simulink model "sampleModel20"  (R2021a)
settings: Solver=VariableStepAuto  StartTime=0.0  StopTime=10.0  RelTol=1e-3
undefined symbols (not defined in the file): DiscIntNeverNeededParam, magnitude, Newton, Raphson
libraries: simulink x274, pid_lib x17
(part 7 of 16)

== system sampleModel20/cfblk93/cfblk6/cfblk8 ==
  cfblk1 : Inport
  cfblk5 : Inport  Port=2
  cfblk6 : Inport  Port=3
  cfblk7 : Inport  Port=4
  cfblk8 : Inport  Port=5
  cfblk9 : Inport  Port=6
  cfblk10 : Inport  Port=7
  cfblk3 : Math  Operator=hypot  SaturateOnIntegerOverflow=on
  cfblk4 : Sin  TimeSource=Use external signal  SampleTime=0
  cfblk2 : Outport
  wires:
  cfblk9/1 -> cfblk3/1
  cfblk1/1 -> cfblk3/2
  cfblk6/1 -> cfblk4/1
  cfblk10/1 -> cfblk2/1

== system sampleModel20/cfblk93/cfblk6/cfblk9 ==
  cfblk1 : Inport
  cfblk13 : Inport  Port=2
  cfblk14 : Inport  Port=3
  cfblk15 : Inport  Port=4
  cfblk16 : Inport  Port=5
  cfblk10 : Bias  Bias=[64527003.954944]
  cfblk11 : Subsystem
  cfblk12 : Subsystem
  cfblk17 : Delay  SampleTime=1
  cfblk18 : Delay  SampleTime=1
  cfblk3 : DiscreteIntegrator  ICPrevOutput=DiscIntNeverNeededParam  ICPrevScaledInput=DiscIntNeverNeededParam
  cfblk4 : Polyval  Coefs=[ +2.081618890e-019, -1.441693666e-014, +4.719686976e-010, -8.536869453e-006, +1.621573104e-001, -8.087801117e+001 ]
  cfblk5 : UnaryMinus
  cfblk6 : Polyval  Coefs=[ +2.081618890e-019, -1.441693666e-014, +4.719686976e-010, -8.536869453e-006, +1.621573104e-001, -8.087801117e+001 ]
  cfblk7 : Trigonometry
  cfblk8 : Math  Operator=mod  SaturateOnIntegerOverflow=on
  cfblk9 : MinMax  Function=max  Inputs=2
  cfblk2 : Outport
  wires:
  cfblk7/1 -> cfblk8/1
  cfblk10/1 -> cfblk7/1
  cfblk6/1 -> cfblk9/1
  cfblk8/1 -> cfblk3/1
  cfblk12/1(cfblk2) -> cfblk4/1
  cfblk13/1 -> cfblk5/1
  cfblk5/1 -> cfblk12/1(cfblk1)
  cfblk11/1(cfblk2) -> cfblk12/2(cfblk11)
  cfblk14/1 -> cfblk9/2, cfblk12/7(cfblk16)
  cfblk3/1 -> cfblk2/1, cfblk12/4(cfblk13)
  cfblk15/1 -> cfblk8/2, cfblk11/4(cfblk6)
  cfblk11/2(cfblk7) -> cfblk10/1, cfblk12/3(cfblk12)
  cfblk16/1 -> cfblk11/2(cfblk4), cfblk12/5(cfblk14), cfblk12/6(cfblk15)
  cfblk1/1 -> cfblk11/3(cfblk5)
  cfblk4/1 -> cfblk17/1
  cfblk17/1 -> cfblk11/1(cfblk1)
  cfblk9/1 -> cfblk18/1
  cfblk18/1 -> cfblk6/1

== system sampleModel20/cfblk93/cfblk7/cfblk10 ==
  cfblk1 : Inport
  cfblk6 : Inport  Port=2
  cfblk7 : Inport  Port=3
  cfblk3 : Sum
  cfblk4 : Subsystem
  cfblk5 : Subsystem
  cfblk8 : Delay  SampleTime=1
  cfblk9 : Delay  SampleTime=1
  cfblk2 : Outport
  wires:
  cfblk6/1 -> cfblk4/1(cfblk1), cfblk4/4(cfblk11), cfblk4/5(cfblk12), cfblk5/7(cfblk11)
  cfblk1/1 -> cfblk3/1, cfblk5/4(cfblk8), cfblk5/5(cfblk9)
  cfblk3/1 -> cfblk4/2(cfblk9), cfblk5/6(cfblk10), cfblk4/6(cfblk13)
  cfblk5/1(cfblk2) -> cfblk2/1, cfblk9/1
  cfblk7/1 -> cfblk5/1(cfblk1), cfblk4/7(cfblk14), cfblk4/8(cfblk15)
  cfblk4/2(cfblk16) -> cfblk5/2(cfblk6)
  cfblk4/3(cfblk17) -> cfblk5/3(cfblk7)
  cfblk4/1(cfblk2) -> cfblk8/1
  cfblk8/1 -> cfblk3/2
  cfblk9/1 -> cfblk4/3(cfblk10)

== system sampleModel20/cfblk94/cfblk10/cfblk6 ==
  cfblk1 : Inport
  cfblk6 : Inport  Port=2
  cfblk7 : Inport  Port=3
  cfblk8 : Inport  Port=4
  cfblk9 : Inport  Port=5
  cfblk10 : Inport  Port=6
  cfblk3 : simulink/Discrete/Tapped Delay  vinit=0.0  samptime=-1  NumDelays=1  DelayOrder=Oldest  includeCurrent=off
  cfblk4 : Sqrt  SaturateOnIntegerOverflow=on
  cfblk5 : Subsystem
  cfblk2 : Outport
  cfblk11 : Outport  Port=2
  cfblk12 : Outport  Port=3
  cfblk13 : Outport  Port=4
  wires:
  cfblk6/1 -> cfblk5/1(cfblk1)
  cfblk8/1 -> cfblk12/1
  cfblk3/1 -> cfblk5/2(cfblk5)
  cfblk10/1 -> cfblk13/1
  cfblk9/1 -> cfblk3/1, cfblk5/4(cfblk7)
  cfblk4/1 -> cfblk11/1
  cfblk5/1(cfblk2) -> cfblk2/1
  cfblk7/1 -> cfblk4/1
  cfblk1/1 -> cfblk5/3(cfblk6), cfblk5/5(cfblk8)

== system sampleModel20/cfblk94/cfblk10/cfblk7 ==
  cfblk1 : Inport
  cfblk10 : Inport  Port=2
  cfblk11 : Inport  Port=3
  cfblk12 : Inport  Port=4
  cfblk13 : Inport  Port=5
  cfblk{15..26} (12 alike) : Delay  SampleTime=1
  cfblk3 : ComplexToMagnitudeAngle
  cfblk4 : Subsystem
  cfblk5 : Subsystem
  cfblk6 : Subsystem
  cfblk7 : Subsystem
  cfblk8 : Subsystem
  cfblk9 : Subsystem
  cfblk2 : Outport
  cfblk14 : Outport  Port=2
  wires:
  cfblk1/1 -> cfblk8/1(cfblk1), cfblk4/5(cfblk10)
  cfblk8/1(cfblk2) -> cfblk5/1(cfblk1)
  cfblk6/1(cfblk2) -> cfblk2/1
  cfblk9/1(cfblk2) -> cfblk3/1
  cfblk12/1 -> cfblk9/2(cfblk10), cfblk7/6(cfblk14)
  cfblk13/1 -> cfblk5/2(cfblk11), cfblk6/4(cfblk12), cfblk8/7(cfblk9), cfblk7/8(cfblk16)
  cfblk3/2 -> cfblk4/8(cfblk13), cfblk16/1, cfblk17/1, cfblk18/1, cfblk19/1
  cfblk8/2(cfblk10) -> cfblk7/1(cfblk1)
  cfblk11/1 -> cfblk7/3(cfblk11), cfblk4/1(cfblk1), cfblk4/2(cfblk7), cfblk7/5(cfblk13), cfblk4/6(cfblk11)
  cfblk4/1(cfblk2) -> cfblk14/1
  cfblk9/3(cfblk17) -> cfblk21/1, cfblk22/1, cfblk23/1
  cfblk8/3(cfblk11) -> cfblk5/3(cfblk12)
  cfblk7/1(cfblk2) -> cfblk6/1(cfblk1)
  cfblk7/2(cfblk17) -> cfblk6/2(cfblk10), cfblk4/9(cfblk14), cfblk24/1, cfblk25/1
  cfblk10/1 -> cfblk5/4(cfblk13)
  cfblk6/2(cfblk14) -> cfblk9/4(cfblk12), cfblk4/3(cfblk8), cfblk9/7(cfblk15)
  cfblk5/1(cfblk2) -> cfblk7/4(cfblk12)
  cfblk5/2(cfblk16) -> cfblk6/3(cfblk11)
  cfblk5/3(cfblk17) -> cfblk9/5(cfblk13), cfblk4/4(cfblk9), cfblk9/6(cfblk14), cfblk4/7(cfblk12), cfblk26/1
  cfblk3/1 -> cfblk15/1
  cfblk15/1 -> cfblk9/1(cfblk1)
  cfblk16/1 -> cfblk9/3(cfblk11)
  cfblk17/1 -> cfblk5/6(cfblk15)
  cfblk18/1 -> cfblk6/5(cfblk13)
  cfblk19/1 -> cfblk7/7(cfblk15)
  cfblk9/2(cfblk16) -> cfblk20/1
  cfblk20/1 -> cfblk7/2(cfblk10)
  cfblk21/1 -> cfblk8/2(cfblk4)
  cfblk22/1 -> cfblk8/3(cfblk5)
  cfblk23/1 -> cfblk8/4(cfblk6)
  cfblk24/1 -> cfblk5/5(cfblk14)
  cfblk25/1 -> cfblk8/6(cfblk8)
  cfblk26/1 -> cfblk8/5(cfblk7)

== system sampleModel20/cfblk94/cfblk11/cfblk6 ==
  cfblk1 : Inport
  cfblk6 : Inport  Port=2
  cfblk7 : Inport  Port=3
  cfblk8 : Inport  Port=4
  cfblk9 : Inport  Port=5
  cfblk10 : Delay  SampleTime=1
  cfblk11 : Delay  SampleTime=1
  cfblk12 : Delay  SampleTime=1
  cfblk3 : Delay  DelayLengthSource=Input port  SampleTime=1
      settings: InputPortMap=u0,p1
  cfblk4 : Subsystem
  cfblk5 : Subsystem
  cfblk2 : Outport
  wires:
  cfblk3/1 -> cfblk5/1(cfblk1)
  cfblk8/1 -> cfblk4/1(cfblk1)
  cfblk6/1 -> cfblk2/1
  cfblk4/1(cfblk2) -> cfblk5/2(cfblk4)
  cfblk1/1 -> cfblk4/3(cfblk10)
  cfblk9/1 -> cfblk3/1, cfblk4/6(cfblk13)
  cfblk4/2(cfblk14) -> cfblk3/2
  cfblk7/1 -> cfblk5/3(cfblk5)
  cfblk4/3(cfblk15) -> cfblk5/4(cfblk6)
  cfblk5/1(cfblk2) -> cfblk10/1
  cfblk10/1 -> cfblk4/2(cfblk9)
  cfblk5/2(cfblk7) -> cfblk11/1
  cfblk11/1 -> cfblk4/4(cfblk11)
  cfblk5/3(cfblk8) -> cfblk12/1
  cfblk12/1 -> cfblk4/5(cfblk12)

== system sampleModel20/cfblk94/cfblk11/cfblk7 ==
  cfblk1 : Inport
  cfblk6 : Inport  Port=2
  cfblk3 : MinMax  Inputs=2
  cfblk4 : Subsystem
  cfblk5 : Subsystem
  cfblk8 : Delay  SampleTime=1
  cfblk9 : Delay  SampleTime=1
  cfblk2 : Outport
  cfblk7 : Outport  Port=2
  wires:
  cfblk3/1 -> cfblk7/1, cfblk5/1(cfblk1), cfblk5/3(cfblk10)
  cfblk6/1 -> cfblk4/1(cfblk1), cfblk5/2(cfblk9)
  cfblk5/1(cfblk2) -> cfblk4/2(cfblk8), cfblk4/4(cfblk10)
  cfblk4/1(cfblk2) -> cfblk8/1, cfblk9/1
  cfblk1/1 -> cfblk2/1, cfblk3/2, cfblk4/3(cfblk9)
  cfblk8/1 -> cfblk3/1
  cfblk9/1 -> cfblk5/4(cfblk11)

== system sampleModel20/cfblk94/cfblk6/cfblk7 ==
  cfblk1 : Inport
  cfblk9 : Inport  Port=2
  cfblk10 : Inport  Port=3
  cfblk11 : Inport  Port=4
  cfblk{12..18} (7 alike) : Delay  SampleTime=1
  cfblk3 : Sin  TimeSource=Use external signal  SampleTime=0
  cfblk4 : Product  Inputs=*
  cfblk5 : Subsystem
  cfblk6 : Subsystem
  cfblk7 : Subsystem
  cfblk8 : Subsystem
  cfblk2 : Outport
  wires:
  cfblk11/1 -> cfblk4/1, cfblk3/1, cfblk8/6(cfblk11), cfblk5/7(cfblk11)
  cfblk1/1 -> cfblk6/1(cfblk1)
  cfblk3/1 -> cfblk7/1(cfblk1), cfblk6/8(cfblk14), cfblk5/6(cfblk10)
  cfblk7/1(cfblk2) -> cfblk2/1
  cfblk9/1 -> cfblk6/2(cfblk8), cfblk5/2(cfblk6), cfblk7/4(cfblk12), cfblk7/6(cfblk14), cfblk7/8(cfblk16)
  cfblk7/2(cfblk17) -> cfblk15/1, cfblk16/1, cfblk17/1, cfblk18/1
  cfblk4/1 -> cfblk7/2(cfblk10), cfblk7/7(cfblk15)
  cfblk6/1(cfblk2) -> cfblk8/3(cfblk8)
  cfblk10/1 -> cfblk6/5(cfblk11), cfblk7/5(cfblk13), cfblk5/4(cfblk8)
  cfblk8/3(cfblk15) -> cfblk5/1(cfblk1), cfblk7/3(cfblk11)
  cfblk6/2(cfblk15) -> cfblk8/4(cfblk9), cfblk5/3(cfblk7), cfblk8/7(cfblk12), cfblk8/8(cfblk13), cfblk5/5(cfblk9)
  cfblk8/1(cfblk2) -> cfblk12/1
  cfblk12/1 -> cfblk6/3(cfblk9)
  cfblk8/2(cfblk14) -> cfblk13/1
  cfblk13/1 -> cfblk6/4(cfblk10)
  cfblk5/1(cfblk2) -> cfblk14/1
  cfblk14/1 -> cfblk8/1(cfblk1)
  cfblk15/1 -> cfblk8/2(cfblk7)
  cfblk16/1 -> cfblk6/6(cfblk12)
  cfblk17/1 -> cfblk8/5(cfblk10)
  cfblk18/1 -> cfblk6/7(cfblk13)

== system sampleModel20/cfblk94/cfblk6/cfblk8 ==
  cfblk1 : Inport
  cfblk9 : Inport  Port=2
  cfblk10 : Inport  Port=3
  cfblk11 : Inport  Port=4
  cfblk12 : Inport  Port=5
  cfblk13 : Inport  Port=6
  cfblk{14..23} (10 alike) : Delay  SampleTime=1
  cfblk3 : Assignment  DiagnosticForDimensions=Warning  IndexOptions=Index vector (dialog)  Indices=1  OutputSizes=1
  cfblk4 : Assignment  DiagnosticForDimensions=Warning  IndexOptions=Index vector (dialog)  Indices=1  OutputSizes=1
  cfblk5 : Subsystem
  cfblk6 : Subsystem
  cfblk7 : Subsystem
  cfblk8 : Subsystem
  cfblk2 : Outport
  wires:
  cfblk9/1 -> cfblk4/1
  cfblk3/1 -> cfblk2/1, cfblk15/1, cfblk16/1
  cfblk12/1 -> cfblk4/2, cfblk6/7(cfblk14), cfblk8/6(cfblk10)
  cfblk4/1 -> cfblk6/1(cfblk1)
  cfblk13/1 -> cfblk7/1(cfblk1), cfblk7/2(cfblk9)
  cfblk8/1(cfblk2) -> cfblk5/1(cfblk1)
  cfblk10/1 -> cfblk5/2(cfblk9)
  cfblk11/1 -> cfblk3/1, cfblk7/3(cfblk10), cfblk7/4(cfblk11)
  cfblk1/1 -> cfblk8/2(cfblk6), cfblk8/4(cfblk8), cfblk5/8(cfblk15), cfblk7/6(cfblk13)
  cfblk7/4(cfblk16) -> cfblk21/1, cfblk22/1
  cfblk6/1(cfblk2) -> cfblk3/2
  cfblk8/2(cfblk11) -> cfblk6/4(cfblk11)
  cfblk5/2(cfblk16) -> cfblk6/5(cfblk12), cfblk6/6(cfblk13), cfblk23/1
  cfblk6/2(cfblk15) -> cfblk7/5(cfblk12), cfblk17/1
  cfblk5/1(cfblk2) -> cfblk14/1
  cfblk14/1 -> cfblk8/3(cfblk7)
  cfblk15/1 -> cfblk5/5(cfblk12)
  cfblk16/1 -> cfblk5/7(cfblk14)
  cfblk17/1 -> cfblk5/4(cfblk11)
  cfblk7/1(cfblk2) -> cfblk18/1
  cfblk18/1 -> cfblk6/2(cfblk9)
  cfblk7/2(cfblk14) -> cfblk19/1
  cfblk19/1 -> cfblk6/3(cfblk10)
  cfblk7/3(cfblk15) -> cfblk20/1
  cfblk20/1 -> cfblk8/1(cfblk1)
  cfblk21/1 -> cfblk5/3(cfblk10)
  cfblk22/1 -> cfblk5/6(cfblk13)
  cfblk23/1 -> cfblk8/5(cfblk9)

== system sampleModel20/cfblk94/cfblk7/cfblk4 ==
  cfblk1 : Inport
  cfblk10 : Inport  Port=2
  cfblk11 : Inport  Port=3
  cfblk{13..18} (6 alike) : Delay  SampleTime=1
  cfblk3 : Product  Inputs=**
  cfblk4 : Polyval  Coefs=[ +2.081618890e-019, -1.441693666e-014, +4.719686976e-010, -8.536869453e-006, +1.621573104e-001, -8.087801117e+001 ]
  cfblk5 : Subsystem
  cfblk6 : Subsystem
  cfblk7 : Subsystem
  cfblk8 : Subsystem
  cfblk9 : Subsystem
  cfblk2 : Outport
  cfblk12 : Outport  Port=2
  wires:
  cfblk3/1 -> cfblk8/5(cfblk7), cfblk18/1
  cfblk9/1(cfblk2) -> cfblk4/1, cfblk8/2(cfblk4), cfblk8/3(cfblk5), cfblk2/1, cfblk7/2(cfblk7)
  cfblk10/1 -> cfblk3/1, cfblk8/8(cfblk10)
  cfblk1/1 -> cfblk6/3(cfblk12)
  cfblk7/1(cfblk2) -> cfblk5/1(cfblk1)
  cfblk6/1(cfblk2) -> cfblk9/1(cfblk1)
  cfblk8/2(cfblk11) -> cfblk7/1(cfblk1)
  cfblk6/2(cfblk17) -> cfblk3/2, cfblk7/3(cfblk8), cfblk7/4(cfblk9), cfblk8/4(cfblk6), cfblk8/6(cfblk8), cfblk8/7(cfblk9)
  cfblk11/1 -> cfblk9/3(cfblk9), cfblk6/7(cfblk16)
  cfblk5/2(cfblk8) -> cfblk12/1
  cfblk7/3(cfblk11) -> cfblk5/2(cfblk7), cfblk16/1
  cfblk4/1 -> cfblk8/1(cfblk1)
  cfblk8/1(cfblk2) -> cfblk13/1
  cfblk13/1 -> cfblk6/2(cfblk11)
  cfblk5/1(cfblk2) -> cfblk14/1
  cfblk14/1 -> cfblk6/4(cfblk13)
  cfblk7/2(cfblk10) -> cfblk15/1
  cfblk15/1 -> cfblk9/2(cfblk8)
  cfblk16/1 -> cfblk6/5(cfblk14)
  cfblk8/3(cfblk12) -> cfblk17/1
  cfblk17/1 -> cfblk6/6(cfblk15)
  cfblk18/1 -> cfblk6/1(cfblk1)

== system sampleModel20/cfblk94/cfblk8/cfblk8 ==
  cfblk1 : Inport
  cfblk8 : Inport  Port=2
  cfblk9 : Inport  Port=3
  cfblk11 : Delay  SampleTime=1
  cfblk3 : Sum  Inputs=+
  cfblk4 : Sum  Inputs=+
  cfblk5 : MinMax  Function=max
  cfblk6 : Subsystem
  cfblk7 : Subsystem
  cfblk2 : Outport
  cfblk10 : Outport  Port=2
  wires:
  cfblk6/1(cfblk2) -> cfblk5/1, cfblk7/4(cfblk9), cfblk7/7(cfblk12)
  cfblk5/1 -> cfblk7/1(cfblk1)
  cfblk9/1 -> cfblk3/1
  cfblk4/1 -> cfblk2/1, cfblk11/1
  cfblk3/1 -> cfblk7/2(cfblk7), cfblk6/3(cfblk12), cfblk7/5(cfblk10), cfblk10/1, cfblk7/6(cfblk11)
  cfblk1/1 -> cfblk6/2(cfblk11)
  cfblk8/1 -> cfblk7/3(cfblk8)
  cfblk7/1(cfblk2) -> cfblk4/1
  cfblk11/1 -> cfblk6/1(cfblk1)

== system sampleModel20/cfblk94/cfblk8/cfblk9 ==
  cfblk1 : Inport
  cfblk6 : Inport  Port=2
  cfblk7 : Inport  Port=3
  cfblk8 : Inport  Port=4
  cfblk3 : Squeeze
  cfblk4 : simulink/Math Operations/MinMax Running Resettable  Function=min  vinit=0.0
  cfblk5 : Subsystem
  cfblk2 : Outport
  cfblk9 : Outport  Port=2
  wires:
  cfblk1/1 -> cfblk5/1(cfblk1)
  cfblk3/1 -> cfblk5/2(cfblk6), cfblk5/5(cfblk9)
  cfblk6/1 -> cfblk4/1, cfblk5/3(cfblk7)
  cfblk8/1 -> cfblk4/2
  cfblk7/1 -> cfblk2/1
  cfblk5/1(cfblk2) -> cfblk9/1
  cfblk4/1 -> cfblk3/1, cfblk5/4(cfblk8), cfblk5/6(cfblk10)

== system sampleModel20/cfblk94/cfblk9/cfblk6 ==
  cfblk1 : Inport
  cfblk11 : Inport  Port=2
  cfblk12 : Inport  Port=3
  cfblk10 : Subsystem
  cfblk{15..21} (7 alike) : Delay  SampleTime=1
  cfblk3 : Gain  Gain=[597722013.813151]
  cfblk4 : Gain  Gain=[-468579084.699582]
  cfblk5 : simulink/Math Operations/Slider Gain  gain=1  low=0  high=2
  cfblk6 : ComplexToMagnitudeAngle
  cfblk7 : DotProduct  InputSameDT=on  OutDataTypeStr=Inherit: Inherit via internal rule
  cfblk8 : Subsystem
  cfblk9 : Subsystem
  cfblk2 : Outport
  cfblk13 : Outport  Port=2
  cfblk14 : Outport  Port=3
  wires:
  cfblk3/1 -> cfblk5/1, cfblk10/5(cfblk6), cfblk10/8(cfblk9)
  cfblk10/1(cfblk2) -> cfblk13/1
  cfblk11/1 -> cfblk6/1, cfblk10/2(cfblk3), cfblk10/4(cfblk5)
  cfblk5/1 -> cfblk2/1, cfblk10/3(cfblk4), cfblk15/1
  cfblk6/1 -> cfblk9/1(cfblk1)
  cfblk10/2(cfblk12) -> cfblk7/2
  cfblk8/1(cfblk2) -> cfblk3/1
  cfblk10/3(cfblk13) -> cfblk14/1
  cfblk12/1 -> cfblk8/2(cfblk9)
  cfblk6/2 -> cfblk9/2(cfblk7)
  cfblk7/1 -> cfblk9/3(cfblk8), cfblk20/1
  cfblk1/1 -> cfblk8/3(cfblk10), cfblk10/6(cfblk7), cfblk10/7(cfblk8)
  cfblk9/1(cfblk2) -> cfblk4/1
  cfblk8/2(cfblk13) -> cfblk9/4(cfblk9)
  cfblk9/3(cfblk11) -> cfblk18/1, cfblk19/1
  cfblk15/1 -> cfblk8/5(cfblk12)
  cfblk4/1 -> cfblk16/1
  cfblk16/1 -> cfblk7/1
  cfblk9/2(cfblk10) -> cfblk17/1
  cfblk17/1 -> cfblk10/1(cfblk1)
  cfblk18/1 -> cfblk8/4(cfblk11)
  cfblk19/1 -> cfblk10/9(cfblk10)
  cfblk20/1 -> cfblk10/10(cfblk11)
  cfblk10/4(cfblk14) -> cfblk21/1
  cfblk21/1 -> cfblk8/1(cfblk1)

== system sampleModel20/cfblk95/cfblk10/cfblk7 ==
  cfblk1 : Inport
  cfblk10 : Delay  SampleTime=1
  cfblk11 : Delay  SampleTime=1
  cfblk3 : PermuteDimensions
  cfblk4 : Bias  Bias=[82997727.223384]
  cfblk5 : Sqrt  SaturateOnIntegerOverflow=on
  cfblk6 : ComplexToRealImag
  cfblk7 : Subsystem
  cfblk8 : Subsystem
  cfblk9 : Subsystem
  cfblk2 : Outport
  wires:
  cfblk5/1 -> cfblk9/1(cfblk1)
  cfblk7/1(cfblk2) -> cfblk2/1
  cfblk1/1 -> cfblk6/1, cfblk4/1, cfblk9/4(cfblk10)
  cfblk3/1 -> cfblk7/1(cfblk1)
  cfblk9/1(cfblk2) -> cfblk7/2(cfblk7)
  cfblk8/1(cfblk2) -> cfblk3/1, cfblk9/2(cfblk8), cfblk9/3(cfblk9)
  cfblk9/2(cfblk12) -> cfblk10/1, cfblk11/1
  cfblk4/1 -> cfblk8/2(cfblk6)
  cfblk6/1 -> cfblk8/3(cfblk7)
  cfblk6/2 -> cfblk5/1, cfblk9/5(cfblk11), cfblk8/5(cfblk9)
  cfblk10/1 -> cfblk8/1(cfblk1)
  cfblk11/1 -> cfblk8/4(cfblk8)

== system sampleModel20/cfblk95/cfblk11/cfblk5 ==
  cfblk1 : Inport
  cfblk10 : Inport  Port=2
  cfblk11 : Inport  Port=3
  cfblk12 : Inport  Port=4
  cfblk13 : Inport  Port=5
  cfblk14 : Inport  Port=6
  cfblk{15..20} (6 alike) : Delay  SampleTime=1
  cfblk3 : Trigonometry
  cfblk4 : Sqrt  Operator=rSqrt  AlgorithmType=Newton-Raphson  SaturateOnIntegerOverflow=on
  cfblk5 : Sum  Inputs=-+
  cfblk6 : Bias  Bias=[930248556.439330]
  cfblk7 : Subsystem
  cfblk8 : Subsystem
  cfblk9 : Subsystem
  cfblk2 : Outport
  wires:
  cfblk14/1 -> cfblk8/1(cfblk1)
  cfblk5/1 -> cfblk8/4(cfblk11), cfblk20/1
  cfblk11/1 -> cfblk2/1
  cfblk1/1 -> cfblk4/1, cfblk8/6(cfblk13)
  cfblk3/1 -> cfblk5/1
  cfblk13/1 -> cfblk5/2
  cfblk12/1 -> cfblk7/1(cfblk1)
  cfblk9/1(cfblk2) -> cfblk6/1
  cfblk9/2(cfblk12) -> cfblk7/3(cfblk8), cfblk8/2(cfblk9)
  cfblk4/1 -> cfblk9/4(cfblk10), cfblk8/3(cfblk10)
  cfblk10/1 -> cfblk7/4(cfblk9)
  cfblk7/1(cfblk2) -> cfblk8/5(cfblk12), cfblk16/1
  cfblk6/1 -> cfblk15/1
  cfblk15/1 -> cfblk9/3(cfblk9)
  cfblk16/1 -> cfblk9/5(cfblk11)
  cfblk8/1(cfblk2) -> cfblk17/1
  cfblk17/1 -> cfblk9/1(cfblk1)
  cfblk8/2(cfblk14) -> cfblk18/1
  cfblk18/1 -> cfblk7/2(cfblk7)
  cfblk8/3(cfblk15) -> cfblk19/1
  cfblk19/1 -> cfblk9/2(cfblk8)
  cfblk20/1 -> cfblk3/1

== system sampleModel20/cfblk95/cfblk11/cfblk6 ==
  cfblk1 : Inport
  cfblk5 : Inport  Port=2
  cfblk6 : Inport  Port=3
  cfblk7 : Inport  Port=4
  cfblk8 : Inport  Port=5
  cfblk11 : Delay  SampleTime=1
  cfblk3 : Subsystem
  cfblk4 : Subsystem
  cfblk2 : Outport
  cfblk9 : Outport  Port=2
  cfblk10 : Outport  Port=3
  wires:
  cfblk3/1(cfblk2) -> cfblk10/1
  cfblk6/1 -> cfblk9/1
  cfblk1/1 -> cfblk4/1(cfblk1)
  cfblk7/1 -> cfblk4/2(cfblk7)
  cfblk5/1 -> cfblk4/3(cfblk8)
  cfblk8/1 -> cfblk4/4(cfblk9)
  cfblk4/1(cfblk2) -> cfblk3/1(cfblk1)
  cfblk4/2(cfblk11) -> cfblk3/2(cfblk9)
  cfblk4/3(cfblk12) -> cfblk2/1
  cfblk3/2(cfblk10) -> cfblk11/1
  cfblk11/1 -> cfblk4/5(cfblk10)

== system sampleModel20/cfblk95/cfblk6/cfblk5 ==
  cfblk1 : Inport
  cfblk11 : Inport  Port=2
  cfblk12 : Inport  Port=3
  cfblk13 : Inport  Port=4
  cfblk14 : Inport  Port=5
  cfblk10 : Subsystem
  cfblk{16..26} (11 alike) : Delay  SampleTime=1
  cfblk3 : ComplexToMagnitudeAngle
  cfblk4 : Abs
  cfblk5 : Assignment  DiagnosticForDimensions=Warning  IndexOptions=Index vector (dialog)  Indices=1  OutputSizes=1
  cfblk6 : Sqrt  Operator=rSqrt  AlgorithmType=Newton-Raphson  SaturateOnIntegerOverflow=on
  cfblk7 : Product  Inputs=**
  cfblk8 : Subsystem
  cfblk9 : Subsystem
  cfblk2 : Outport
  cfblk15 : Outport  Port=2
  wires:
  cfblk5/1 -> cfblk3/1, cfblk24/1
  cfblk14/1 -> cfblk15/1, cfblk9/7(cfblk15)
  cfblk1/1 -> cfblk4/1
  cfblk3/1 -> cfblk6/1
  cfblk9/1(cfblk2) -> cfblk10/1(cfblk1)
  cfblk13/1 -> cfblk2/1
  cfblk7/1 -> cfblk5/1
  cfblk8/1(cfblk2) -> cfblk9/1(cfblk1)
  cfblk4/1 -> cfblk8/1(cfblk1), cfblk8/8(cfblk16)
  cfblk11/1 -> cfblk9/2(cfblk10)
  cfblk8/2(cfblk17) -> cfblk10/2(cfblk8)
  cfblk9/2(cfblk16) -> cfblk10/3(cfblk9)
  cfblk12/1 -> cfblk5/2
  cfblk6/1 -> cfblk21/1, cfblk22/1
  cfblk10/6(cfblk14) -> cfblk7/2, cfblk25/1
  cfblk10/1(cfblk2) -> cfblk16/1
  cfblk16/1 -> cfblk9/3(cfblk11)
  cfblk10/2(cfblk10) -> cfblk17/1
  cfblk17/1 -> cfblk9/4(cfblk12)
  cfblk10/3(cfblk11) -> cfblk18/1
  cfblk18/1 -> cfblk8/3(cfblk11)
  cfblk10/4(cfblk12) -> cfblk19/1
  cfblk19/1 -> cfblk8/4(cfblk12)
  cfblk10/5(cfblk13) -> cfblk20/1
  cfblk20/1 -> cfblk8/5(cfblk13)
  cfblk21/1 -> cfblk9/5(cfblk13)
  cfblk22/1 -> cfblk8/6(cfblk14)
  cfblk3/2 -> cfblk23/1
  cfblk23/1 -> cfblk7/1
  cfblk24/1 -> cfblk8/7(cfblk15)
  cfblk25/1 -> cfblk9/6(cfblk14)
  cfblk9/3(cfblk17) -> cfblk26/1
  cfblk26/1 -> cfblk8/2(cfblk10)

== system sampleModel20/cfblk95/cfblk6/cfblk6 ==
  cfblk1 : Inport
  cfblk11 : Inport  Port=2
  cfblk12 : Inport  Port=3
  cfblk10 : Subsystem
  cfblk{15..20} (6 alike) : Delay  SampleTime=1
  cfblk3 : Assignment  DiagnosticForDimensions=Warning  IndexOptions=Index vector (dialog)  Indices=1  OutputSizes=1
  cfblk4 : simulink/Math Operations/MinMax Running Resettable  Function=min  vinit=0.0
  cfblk5 : Rounding
  cfblk6 : Signum
  cfblk7 : ComplexToRealImag
  cfblk8 : Subsystem
  cfblk9 : Subsystem
  cfblk2 : Outport
  cfblk13 : Outport  Port=2
  cfblk14 : Outport  Port=3
  wires:
  cfblk8/1(cfblk2) -> cfblk10/1(cfblk1), cfblk14/1
  cfblk10/1(cfblk2) -> cfblk4/1
  cfblk1/1 -> cfblk7/1, cfblk8/3(cfblk8)
  cfblk10/2(cfblk11) -> cfblk5/1
  cfblk9/1(cfblk2) -> cfblk3/1
  cfblk11/1 -> cfblk9/1(cfblk1)
  cfblk9/2(cfblk13) -> cfblk17/1, cfblk18/1
  cfblk12/1 -> cfblk3/2, cfblk10/4(cfblk8)
  cfblk3/1 -> cfblk4/2, cfblk16/1
  cfblk7/1 -> cfblk2/1
  cfblk7/2 -> cfblk8/2(cfblk7), cfblk9/4(cfblk11), cfblk8/4(cfblk9)
  cfblk5/1 -> cfblk6/1, cfblk9/5(cfblk12), cfblk13/1, cfblk20/1
  cfblk6/1 -> cfblk9/3(cfblk10), cfblk19/1
  cfblk4/1 -> cfblk15/1
  cfblk15/1 -> cfblk10/2(cfblk6)
  cfblk16/1 -> cfblk9/2(cfblk9)
  cfblk17/1 -> cfblk8/1(cfblk1)
  cfblk18/1 -> cfblk10/3(cfblk7)
  cfblk19/1 -> cfblk10/5(cfblk9)
  cfblk20/1 -> cfblk10/6(cfblk10)

== system sampleModel20/cfblk95/cfblk6/cfblk7 ==
  cfblk1 : Inport
  cfblk12 : Inport  Port=2
  cfblk13 : Inport  Port=3
  cfblk14 : Inport  Port=4
  cfblk15 : Inport  Port=5
  cfblk16 : Inport  Port=6
  cfblk10 : Subsystem
  cfblk11 : Subsystem
  cfblk{17..22} (6 alike) : Delay  SampleTime=1
  cfblk3 : UnaryMinus
  cfblk4 : Sum  Inputs=|++
  cfblk5 : Rounding
  cfblk6 : DotProduct  InputSameDT=on  OutDataTypeStr=Inherit: Inherit via internal rule
  cfblk7 : UnaryMinus
  cfblk8 : simulink/Math Operations/Slider Gain  gain=1  low=0  high=2
  cfblk9 : Subsystem
  cfblk2 : Outport
  wires:
  cfblk9/1(cfblk2) -> cfblk7/1
  cfblk15/1 -> cfblk11/1(cfblk1)
  cfblk12/1 -> cfblk3/1
  cfblk8/1 -> cfblk2/1
  cfblk6/1 -> cfblk18/1, cfblk19/1
  cfblk16/1 -> cfblk11/2(cfblk5), cfblk11/3(cfblk6), cfblk11/4(cfblk7)
  cfblk3/1 -> cfblk9/1(cfblk1), cfblk10/5(cfblk13)
  cfblk14/1 -> cfblk6/1, cfblk9/4(cfblk7)
  cfblk10/1(cfblk2) -> cfblk5/1
  cfblk7/1 -> cfblk4/2
  cfblk13/1 -> cfblk10/1(cfblk1), cfblk11/6(cfblk9)
  cfblk4/1 -> cfblk11/5(cfblk8), cfblk17/1, cfblk21/1, cfblk22/1
  cfblk5/1 -> cfblk9/3(cfblk6)
  cfblk10/2(cfblk16) -> cfblk8/1
  cfblk11/1(cfblk2) -> cfblk6/2
  cfblk1/1 -> cfblk10/2(cfblk10)
  cfblk17/1 -> cfblk9/2(cfblk5)
  cfblk18/1 -> cfblk4/1
  cfblk19/1 -> cfblk10/6(cfblk14)
  cfblk11/2(cfblk10) -> cfblk20/1
  cfblk20/1 -> cfblk10/3(cfblk11)
  cfblk21/1 -> cfblk10/4(cfblk12)
  cfblk22/1 -> cfblk10/7(cfblk15)

== system sampleModel20/cfblk95/cfblk7/cfblk4 ==
  cfblk1 : Inport
  cfblk11 : Inport  Port=2
  cfblk10 : Subsystem
  cfblk{12..21} (10 alike) : Delay  SampleTime=1
  cfblk3 : Signum
  cfblk4 : simulink/Math Operations/MinMax Running Resettable  Function=min  vinit=0.0
  cfblk5 : Assignment  DiagnosticForDimensions=Warning  IndexOptions=Index vector (dialog)  Indices=1  OutputSizes=1
  cfblk6 : Rounding
  cfblk7 : Subsystem
  cfblk8 : Subsystem
  cfblk9 : Subsystem
  cfblk2 : Outport
  wires:
  cfblk10/1(cfblk2) -> cfblk7/1(cfblk1)
  cfblk1/1 -> cfblk10/2(cfblk8), cfblk8/4(cfblk10), cfblk9/4(cfblk10)
  cfblk10/2(cfblk14) -> cfblk3/1
  cfblk9/2(cfblk16) -> cfblk5/1
  cfblk11/1 -> cfblk8/1(cfblk1), cfblk9/3(cfblk9), cfblk9/6(cfblk12)
  cfblk6/1 -> cfblk7/4(cfblk9), cfblk21/1
  cfblk7/1(cfblk2) -> cfblk9/5(cfblk11), cfblk12/1
  cfblk5/1 -> cfblk8/2(cfblk8), cfblk18/1, cfblk19/1
  cfblk10/3(cfblk15) -> cfblk4/1
  cfblk10/4(cfblk16) -> cfblk5/2
  cfblk8/1(cfblk2) -> cfblk2/1
  cfblk4/1 -> cfblk14/1, cfblk15/1
  cfblk10/5(cfblk17) -> cfblk6/1, cfblk7/2(cfblk7), cfblk7/6(cfblk11), cfblk9/8(cfblk14)
  cfblk3/1 -> cfblk8/3(cfblk9), cfblk7/3(cfblk8), cfblk9/7(cfblk13)
  cfblk8/2(cfblk11) -> cfblk4/2, cfblk16/1, cfblk17/1
  cfblk12/1 -> cfblk10/5(cfblk11)
  cfblk9/1(cfblk2) -> cfblk13/1
  cfblk13/1 -> cfblk10/1(cfblk1)
  cfblk14/1 -> cfblk10/6(cfblk12)
  cfblk15/1 -> cfblk10/7(cfblk13)
  cfblk16/1 -> cfblk9/2(cfblk8)
  cfblk17/1 -> cfblk9/9(cfblk15)
  cfblk18/1 -> cfblk9/1(cfblk1)
  cfblk19/1 -> cfblk7/5(cfblk10)
  cfblk9/3(cfblk17) -> cfblk20/1
  cfblk20/1 -> cfblk10/4(cfblk10)
  cfblk21/1 -> cfblk10/3(cfblk9)

== system sampleModel20/cfblk95/cfblk7/cfblk5 ==
  cfblk1 : Inport
  cfblk7 : Inport  Port=2
  cfblk8 : Inport  Port=3
  cfblk9 : Inport  Port=4
  cfblk10 : Inport  Port=5
  cfblk12 : Delay  SampleTime=1
  cfblk13 : Delay  SampleTime=1
  cfblk14 : Delay  SampleTime=1
  cfblk3 : PermuteDimensions
  cfblk4 : Sum  Inputs=|++
  cfblk5 : Subsystem
  cfblk6 : Subsystem
  cfblk2 : Outport
  cfblk11 : Outport  Port=2
  wires:
  cfblk6/1(cfblk2) -> cfblk2/1
  cfblk3/1 -> cfblk5/4(cfblk10), cfblk12/1
  cfblk9/1 -> cfblk6/2(cfblk5)
  cfblk7/1 -> cfblk5/1(cfblk1)
  cfblk4/1 -> cfblk6/3(cfblk6), cfblk5/6(cfblk12)
  cfblk6/2(cfblk8) -> cfblk3/1, cfblk5/5(cfblk11)
  cfblk1/1 -> cfblk4/1, cfblk5/7(cfblk13)
  cfblk8/1 -> cfblk5/2(cfblk8)
  cfblk10/1 -> cfblk5/3(cfblk9)
  cfblk5/3(cfblk15) -> cfblk11/1
  cfblk12/1 -> cfblk6/1(cfblk1)
  cfblk5/1(cfblk2) -> cfblk13/1
  cfblk13/1 -> cfblk6/4(cfblk7)
  cfblk5/2(cfblk14) -> cfblk14/1
  cfblk14/1 -> cfblk4/2

== system sampleModel20/cfblk95/cfblk8/cfblk5 ==
  cfblk1 : Inport
  cfblk7 : Inport  Port=2
  cfblk8 : Inport  Port=3
  cfblk9 : Inport  Port=4
  cfblk10 : Delay  SampleTime=1
  cfblk3 : ComplexToRealImag
  cfblk4 : UnaryMinus
  cfblk5 : Sum  Inputs=|++
  cfblk6 : Subsystem
  cfblk2 : Outport
  wires:
  cfblk3/1 -> cfblk5/1
  cfblk7/1 -> cfblk4/1
  cfblk9/1 -> cfblk6/1(cfblk1)
  cfblk5/1 -> cfblk2/1
  cfblk1/1 -> cfblk6/2(cfblk6)
  cfblk4/1 -> cfblk6/3(cfblk7)
  cfblk6/1(cfblk2) -> cfblk3/1
  cfblk6/2(cfblk9) -> cfblk5/2
  cfblk3/2 -> cfblk10/1
  cfblk10/1 -> cfblk6/4(cfblk8)

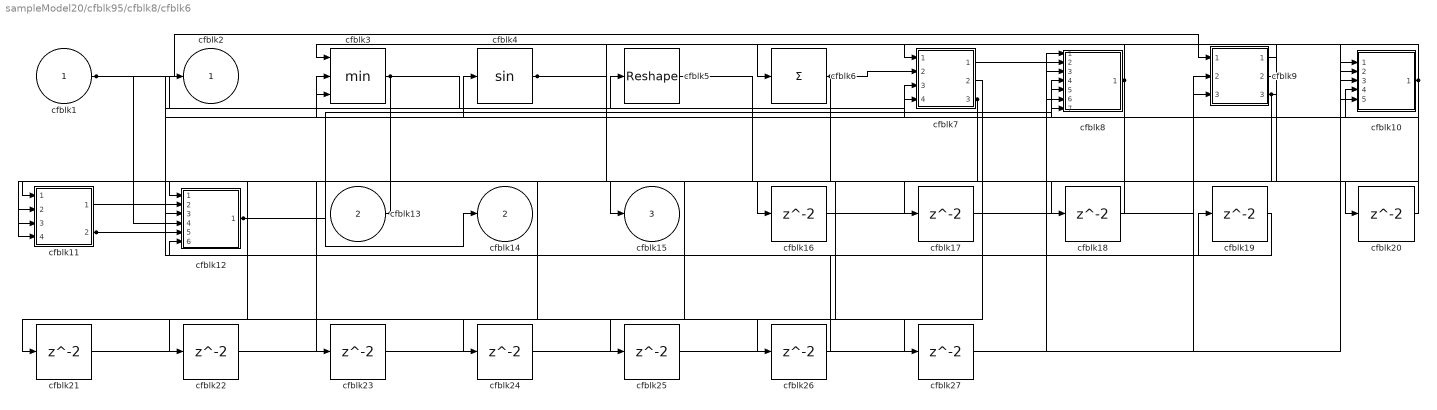
== system sampleModel20/cfblk95/cfblk8/cfblk6 ==
  cfblk1 : Inport
  cfblk13 : Inport  Port=2
  cfblk10 : Subsystem
  cfblk11 : Subsystem
  cfblk12 : Subsystem
  cfblk{16..27} (12 alike) : Delay  SampleTime=1
  cfblk3 : MinMax  Inputs=3
  cfblk4 : Trigonometry
  cfblk5 : Reshape
  cfblk6 : Sum  Inputs=+
  cfblk7 : Subsystem
  cfblk8 : Subsystem
  cfblk9 : Subsystem
  cfblk2 : Outport
  cfblk14 : Outport  Port=2
  cfblk15 : Outport  Port=3
  wires:
  cfblk8/1(cfblk2) -> cfblk6/1, cfblk24/1, cfblk25/1, cfblk26/1, cfblk27/1
  cfblk12/1(cfblk2) -> cfblk14/1, cfblk8/4(cfblk12)
  cfblk1/1 -> cfblk9/1(cfblk1), cfblk10/4(cfblk7), cfblk12/4(cfblk11)
  cfblk9/1(cfblk2) -> cfblk4/1
  cfblk13/1 -> cfblk2/1, cfblk3/3
  cfblk10/1(cfblk2) -> cfblk3/1, cfblk11/4(cfblk6), cfblk12/5(cfblk12)
  cfblk3/1 -> cfblk12/1(cfblk1), cfblk7/4(cfblk7)
  cfblk6/1 -> cfblk11/1(cfblk1), cfblk7/2(cfblk5)
  cfblk11/2(cfblk7) -> cfblk5/1, cfblk19/1
  cfblk4/1 -> cfblk10/2(cfblk5), cfblk8/7(cfblk15), cfblk16/1
  cfblk9/2(cfblk10) -> cfblk15/1
  cfblk9/3(cfblk11) -> cfblk11/3(cfblk5), cfblk3/2, cfblk7/1(cfblk1), cfblk7/3(cfblk6), cfblk12/2(cfblk9), cfblk8/5(cfblk13)
  cfblk7/3(cfblk9) -> cfblk22/1, cfblk23/1
  cfblk16/1 -> cfblk9/2(cfblk8)
  cfblk11/1(cfblk2) -> cfblk17/1
  cfblk17/1 -> cfblk8/1(cfblk1)
  cfblk5/1 -> cfblk18/1
  cfblk18/1 -> cfblk11/2(cfblk4)
  cfblk19/1 -> cfblk12/6(cfblk13)
  cfblk7/1(cfblk2) -> cfblk20/1
  cfblk20/1 -> cfblk8/2(cfblk10)
  cfblk7/2(cfblk8) -> cfblk21/1
  cfblk21/1 -> cfblk9/3(cfblk9)
  cfblk22/1 -> cfblk8/3(cfblk11)
  cfblk23/1 -> cfblk8/6(cfblk14)
  cfblk24/1 -> cfblk10/1(cfblk1)
  cfblk25/1 -> cfblk10/3(cfblk6)
  cfblk26/1 -> cfblk12/3(cfblk10)
  cfblk27/1 -> cfblk10/5(cfblk8)

== system sampleModel20/cfblk95/cfblk8/cfblk7 ==
  cfblk1 : Inport
  cfblk8 : Inport  Port=2
  cfblk9 : Inport  Port=3
  cfblk10 : Inport  Port=4
  cfblk12 : Delay  SampleTime=1
  cfblk13 : Delay  SampleTime=1
  cfblk14 : Delay  SampleTime=1
  cfblk3 : Product  Inputs=*
  cfblk4 : Squeeze
  cfblk5 : Subsystem
  cfblk6 : Subsystem
  cfblk7 : Subsystem
  cfblk2 : Outport
  cfblk11 : Outport  Port=2
  wires:
  cfblk8/1 -> cfblk4/1, cfblk5/6(cfblk10)
  cfblk3/1 -> cfblk2/1, cfblk12/1
  cfblk6/1(cfblk2) -> cfblk7/1(cfblk1)
  cfblk5/1(cfblk2) -> cfblk3/1
  cfblk4/1 -> cfblk7/2(cfblk9)
  cfblk1/1 -> cfblk6/1(cfblk1), cfblk7/4(cfblk11)
  cfblk7/1(cfblk2) -> cfblk5/1(cfblk1)
  cfblk9/1 -> cfblk6/2(cfblk12), cfblk7/6(cfblk13)
  cfblk6/2(cfblk15) -> cfblk11/1
  cfblk10/1 -> cfblk5/2(cfblk6)
  cfblk6/3(cfblk16) -> cfblk7/3(cfblk10), cfblk5/4(cfblk8), cfblk7/5(cfblk12)
  cfblk7/2(cfblk14) -> cfblk5/3(cfblk7)
  cfblk12/1 -> cfblk5/5(cfblk9)
  cfblk7/3(cfblk15) -> cfblk13/1
  cfblk13/1 -> cfblk6/3(cfblk13)
  cfblk7/4(cfblk16) -> cfblk14/1
  cfblk14/1 -> cfblk6/4(cfblk14)

== system sampleModel20/cfblk95/cfblk9/cfblk7 ==
  cfblk1 : Inport
  cfblk{8..11} (4 alike) : Delay  SampleTime=1
  cfblk3 : Rounding
  cfblk4 : Bias  Bias=[-45366030.790602]
  cfblk5 : Reshape
  cfblk6 : Subsystem
  cfblk7 : Subsystem
  cfblk2 : Outport
  wires:
  cfblk5/1 -> cfblk8/1, cfblk9/1, cfblk10/1
  cfblk7/1(cfblk2) -> cfblk4/1, cfblk6/7(cfblk10)
  cfblk4/1 -> cfblk3/1, cfblk6/3(cfblk6), cfblk6/5(cfblk8), cfblk6/8(cfblk11), cfblk6/9(cfblk12)
  cfblk6/1(cfblk2) -> cfblk5/1, cfblk11/1
  cfblk3/1 -> cfblk2/1, cfblk6/1(cfblk1), cfblk6/2(cfblk5), cfblk6/10(cfblk13)
  cfblk1/1 -> cfblk7/2(cfblk6), cfblk6/4(cfblk7), cfblk6/6(cfblk9)
  cfblk8/1 -> cfblk7/1(cfblk1)
  cfblk9/1 -> cfblk7/3(cfblk7)
  cfblk10/1 -> cfblk6/11(cfblk14)
  cfblk11/1 -> cfblk7/4(cfblk8)

== system sampleModel20/cfblk95/cfblk9/cfblk8 ==
  cfblk1 : Inport
  cfblk10 : Delay  SampleTime=1
  cfblk3 : ComplexToMagnitudeAngle
  cfblk4 : Assignment  DiagnosticForDimensions=Warning  IndexOptions=Index vector (dialog)  Indices=1  OutputSizes=1
  cfblk5 : ComplexToRealImag
  cfblk6 : Constant  Value=[-579683967.373903]  SampleTime=1
  cfblk7 : Subsystem
  cfblk8 : Delay  SampleTime=1
  cfblk9 : Delay  SampleTime=1
  cfblk2 : Outport
  wires:
  cfblk5/1 -> cfblk4/1
  cfblk3/1 -> cfblk5/1
  cfblk7/1(cfblk2) -> cfblk4/2
  cfblk7/2(cfblk11) -> cfblk3/1
  cfblk6/1 -> cfblk2/1, cfblk7/5(cfblk10)
  cfblk1/1 -> cfblk7/3(cfblk8)
  cfblk4/1 -> cfblk8/1
  cfblk8/1 -> cfblk7/1(cfblk1)
  cfblk5/2 -> cfblk9/1
  cfblk9/1 -> cfblk7/4(cfblk9)
  cfblk3/2 -> cfblk10/1
  cfblk10/1 -> cfblk7/2(cfblk7)

== system sampleModel20/cfblk96/cfblk5/cfblk4 ==
  cfblk1 : Inport
  cfblk12 : Inport  Port=2
  cfblk10 : Subsystem
  cfblk11 : Subsystem
  cfblk{13..20} (8 alike) : Delay  SampleTime=1
  cfblk3 : Sqrt  SaturateOnIntegerOverflow=on
  cfblk4 : Sum  Inputs=+
  cfblk5 : Sum  Inputs=+
  cfblk6 : MinMax  Inputs=3
  cfblk7 : Abs
  cfblk8 : Sum  Inputs=+-
  cfblk9 : Subsystem
  cfblk2 : Outport
  wires:
  cfblk8/1 -> cfblk5/1, cfblk17/1
  cfblk7/1 -> cfblk3/1
  cfblk1/1 -> cfblk6/1, cfblk10/4(cfblk10)
  cfblk5/1 -> cfblk7/1
  cfblk10/1(cfblk2) -> cfblk2/1
  cfblk3/1 -> cfblk11/3(cfblk6), cfblk13/1, cfblk14/1
  cfblk6/1 -> cfblk9/1(cfblk1)
  cfblk12/1 -> cfblk8/1
  cfblk11/1(cfblk2) -> cfblk4/1
  cfblk10/2(cfblk12) -> cfblk8/2
  cfblk9/1(cfblk2) -> cfblk10/2(cfblk8)
  cfblk10/4(cfblk14) -> cfblk11/1(cfblk1)
  cfblk10/5(cfblk15) -> cfblk11/2(cfblk5)
  cfblk10/6(cfblk16) -> cfblk19/1, cfblk20/1
  cfblk13/1 -> cfblk10/1(cfblk1)
  cfblk14/1 -> cfblk6/2
  cfblk4/1 -> cfblk15/1
  cfblk15/1 -> cfblk10/3(cfblk9)
  cfblk11/2(cfblk7) -> cfblk16/1
  cfblk16/1 -> cfblk9/2(cfblk7)
  cfblk17/1 -> cfblk10/5(cfblk11)
  cfblk10/3(cfblk13) -> cfblk18/1
  cfblk18/1 -> cfblk9/3(cfblk8)
  cfblk19/1 -> cfblk9/4(cfblk9)
  cfblk20/1 -> cfblk6/3

== system sampleModel20/cfblk96/cfblk5/cfblk5 ==
  cfblk1 : Inport
  cfblk7 : Inport  Port=2
  cfblk3 : Product  Inputs=*
  cfblk4 : Sqrt  Operator=rSqrt  AlgorithmType=Newton-Raphson  SaturateOnIntegerOverflow=on
  cfblk5 : Polyval  Coefs=[ +2.081618890e-019, -1.441693666e-014, +4.719686976e-010, -8.536869453e-006, +1.621573104e-001, -8.087801117e+001 ]
  cfblk6 : Abs
  cfblk2 : Outport
  cfblk8 : Outport  Port=2
  wires:
  cfblk6/1 -> cfblk4/1
  cfblk1/1 -> cfblk8/1
  cfblk3/1 -> cfblk5/1
  cfblk5/1 -> cfblk2/1
  cfblk4/1 -> cfblk3/1
  cfblk7/1 -> cfblk6/1

== system sampleModel20/cfblk96/cfblk5/cfblk6 ==
  cfblk1 : Inport
  cfblk8 : Inport  Port=2
  cfblk9 : Inport  Port=3
  cfblk{12..15} (4 alike) : Delay  SampleTime=1
  cfblk3 : simulink/Math Operations/Slider Gain  gain=1  low=0  high=2
  cfblk4 : Signum
  cfblk5 : Subsystem
  cfblk6 : Subsystem
  cfblk7 : Subsystem
  cfblk2 : Outport
  cfblk10 : Outport  Port=2
  cfblk11 : Outport  Port=3
  wires:
  cfblk8/1 -> cfblk6/1(cfblk1), cfblk5/1(cfblk1)
  cfblk7/1(cfblk2) -> cfblk11/1, cfblk5/5(cfblk11)
  cfblk9/1 -> cfblk4/1, cfblk5/2(cfblk8)
  cfblk6/1(cfblk2) -> cfblk3/1, cfblk13/1, cfblk14/1
  cfblk1/1 -> cfblk7/1(cfblk1), cfblk6/4(cfblk11)
  cfblk5/1(cfblk2) -> cfblk6/2(cfblk9)
  cfblk4/1 -> cfblk2/1, cfblk6/5(cfblk12), cfblk6/6(cfblk13), cfblk5/4(cfblk10)
  cfblk3/1 -> cfblk10/1, cfblk12/1
  cfblk5/2(cfblk12) -> cfblk6/3(cfblk10), cfblk6/7(cfblk14), cfblk15/1
  cfblk12/1 -> cfblk7/2(cfblk5)
  cfblk13/1 -> cfblk7/4(cfblk7)
  cfblk14/1 -> cfblk5/3(cfblk9)
  cfblk15/1 -> cfblk7/3(cfblk6)

== system sampleModel20/cfblk96/cfblk5/cfblk7 ==
  cfblk1 : Inport
  cfblk8 : Inport  Port=2
  cfblk9 : Inport  Port=3
  cfblk10 : Inport  Port=4
  cfblk11 : Inport  Port=5
  cfblk12 : Inport  Port=6
  cfblk13 : Inport  Port=7
  cfblk14 : Inport  Port=8
  cfblk15 : Inport  Port=9
  cfblk3 : Gain  Gain=[754065965.765135]
  cfblk4 : Polyval  Coefs=[ +2.081618890e-019, -1.441693666e-014, +4.719686976e-010, -8.536869453e-006, +1.621573104e-001, -8.087801117e+001 ]
  cfblk5 : Sum  Inputs=+-
  cfblk6 : Subsystem
  cfblk7 : Subsystem
  cfblk2 : Outport
  cfblk16 : Outport  Port=2
  wires:
  cfblk8/1 -> cfblk3/1, cfblk6/7(cfblk13), cfblk6/8(cfblk14)
  cfblk6/1(cfblk2) -> cfblk16/1
  cfblk4/1 -> cfblk6/1(cfblk1), cfblk6/5(cfblk11)
  cfblk1/1 -> cfblk4/1
  cfblk14/1 -> cfblk6/2(cfblk8), cfblk6/6(cfblk12)
  cfblk12/1 -> cfblk7/1(cfblk1)
  cfblk3/1 -> cfblk5/1
  cfblk15/1 -> cfblk7/2(cfblk11)
  cfblk9/1 -> cfblk5/2
  cfblk7/1(cfblk2) -> cfblk6/3(cfblk9)
  cfblk10/1 -> cfblk2/1
  cfblk5/1 -> cfblk7/3(cfblk12)
  cfblk11/1 -> cfblk7/4(cfblk13)
  cfblk13/1 -> cfblk7/5(cfblk14), cfblk7/6(cfblk15)
  cfblk7/2(cfblk16) -> cfblk6/4(cfblk10)

== system sampleModel20/cfblk96/cfblk5/cfblk8 ==
  cfblk1 : Inport
  cfblk10 : Inport  Port=2
  cfblk{11..14} (4 alike) : Delay  SampleTime=1
  cfblk3 : simulink/Math Operations/MinMax Running Resettable  Function=min  vinit=0.0
  cfblk4 : Sum  Inputs=+-
  cfblk5 : Product  Inputs=*
  cfblk6 : Subsystem
  cfblk7 : Subsystem
  cfblk8 : Subsystem
  cfblk9 : Subsystem
  cfblk2 : Outport
  wires:
  cfblk6/1(cfblk2) -> cfblk2/1
  cfblk8/1(cfblk2) -> cfblk3/1
  cfblk5/1 -> cfblk6/2(cfblk5), cfblk9/2(cfblk9), cfblk9/4(cfblk11), cfblk9/6(cfblk13)
  cfblk10/1 -> cfblk4/1, cfblk8/4(cfblk13), cfblk7/5(cfblk9)
  cfblk4/1 -> cfblk6/3(cfblk6), cfblk6/7(cfblk10), cfblk5/1, cfblk8/5(cfblk14)
  cfblk6/2(cfblk11) -> cfblk8/1(cfblk1)
  cfblk1/1 -> cfblk4/2, cfblk8/2(cfblk11), cfblk8/3(cfblk12), cfblk9/5(cfblk12)
  cfblk3/1 -> cfblk9/1(cfblk1), cfblk9/7(cfblk14), cfblk7/4(cfblk8)
  cfblk8/3(cfblk16) -> cfblk7/3(cfblk7), cfblk9/3(cfblk10), cfblk14/1
  cfblk6/3(cfblk12) -> cfblk3/2, cfblk9/8(cfblk15)
  cfblk9/1(cfblk2) -> cfblk7/1(cfblk1)
  cfblk9/2(cfblk16) -> cfblk7/2(cfblk6)
  cfblk7/1(cfblk2) -> cfblk11/1
  cfblk11/1 -> cfblk6/1(cfblk1)
  cfblk9/3(cfblk17) -> cfblk12/1
  cfblk12/1 -> cfblk6/6(cfblk9)
  cfblk8/2(cfblk15) -> cfblk13/1
  cfblk13/1 -> cfblk6/4(cfblk7)
  cfblk14/1 -> cfblk6/5(cfblk8)

== system sampleModel20/cfblk96/cfblk6/cfblk5 ==
  cfblk1 : Inport
  cfblk15 : Inport  Port=2
  cfblk10 : Subsystem
  cfblk11 : Subsystem
  cfblk12 : Subsystem
  cfblk13 : Subsystem
  cfblk14 : Subsystem
  cfblk{17..24} (8 alike) : Delay  SampleTime=1
  cfblk3 : Sqrt  SaturateOnIntegerOverflow=on
  cfblk4 : UnaryMinus
  cfblk5 : Rounding
  cfblk6 : Assignment  DiagnosticForDimensions=Warning  IndexOptions=Index vector (dialog)  Indices=1  OutputSizes=1
  cfblk7 : Abs
  cfblk8 : UnaryMinus
  cfblk9 : Sum  Inputs=|++
  cfblk2 : Outport
  cfblk16 : Outport  Port=2
  wires:
  cfblk13/1(cfblk2) -> cfblk14/1(cfblk1)
  cfblk1/1 -> cfblk6/1, cfblk11/6(cfblk9)
  cfblk9/1 -> cfblk3/1
  cfblk7/1 -> cfblk12/3(cfblk7), cfblk24/1
  cfblk6/1 -> cfblk13/2(cfblk7), cfblk14/4(cfblk7), cfblk13/6(cfblk11)
  cfblk3/1 -> cfblk11/2(cfblk5), cfblk20/1, cfblk21/1
  cfblk10/1(cfblk2) -> cfblk12/1(cfblk1), cfblk9/2, cfblk22/1
  cfblk13/2(cfblk12) -> cfblk10/1(cfblk1)
  cfblk11/1(cfblk2) -> cfblk2/1
  cfblk15/1 -> cfblk14/2(cfblk5), cfblk11/5(cfblk8)
  cfblk14/1(cfblk2) -> cfblk5/1, cfblk11/3(cfblk6), cfblk11/4(cfblk7)
  cfblk12/1(cfblk2) -> cfblk11/1(cfblk1)
  cfblk13/3(cfblk13) -> cfblk12/2(cfblk6)
  cfblk4/1 -> cfblk7/1
  cfblk13/4(cfblk14) -> cfblk8/1
  cfblk12/3(cfblk9) -> cfblk16/1, cfblk14/3(cfblk6)
  cfblk13/5(cfblk15) -> cfblk4/1, cfblk11/7(cfblk10)
  cfblk5/1 -> cfblk17/1
  cfblk17/1 -> cfblk13/3(cfblk8)
  cfblk11/2(cfblk11) -> cfblk18/1
  cfblk18/1 -> cfblk6/2
  cfblk12/2(cfblk8) -> cfblk19/1
  cfblk19/1 -> cfblk10/2(cfblk7)
  cfblk20/1 -> cfblk9/1
  cfblk21/1 -> cfblk10/3(cfblk8)
  cfblk22/1 -> cfblk13/5(cfblk10)
  cfblk8/1 -> cfblk23/1
  cfblk23/1 -> cfblk13/4(cfblk9)
  cfblk24/1 -> cfblk13/1(cfblk1)

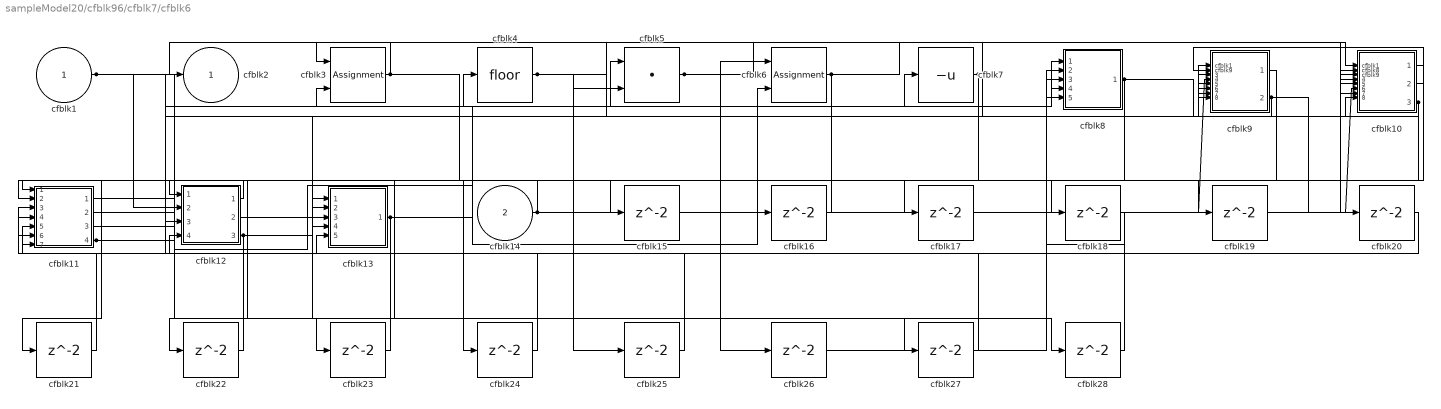
== system sampleModel20/cfblk96/cfblk7/cfblk6 ==
  cfblk1 : Inport
  cfblk14 : Inport  Port=2
  cfblk10 : Subsystem
  cfblk11 : Subsystem
  cfblk12 : Subsystem
  cfblk13 : Subsystem
  cfblk{15..28} (14 alike) : Delay  SampleTime=1
  cfblk3 : Assignment  DiagnosticForDimensions=Warning  IndexOptions=Index vector (dialog)  Indices=1  OutputSizes=1
  cfblk4 : Rounding
  cfblk5 : DotProduct  InputSameDT=on  OutDataTypeStr=Inherit: Inherit via internal rule
  cfblk6 : Assignment  DiagnosticForDimensions=Warning  IndexOptions=Index vector (dialog)  Indices=1  OutputSizes=1
  cfblk7 : UnaryMinus
  cfblk8 : Subsystem
  cfblk9 : Subsystem
  cfblk2 : Outport
  wires:
  cfblk14/1 -> cfblk11/1(cfblk1), cfblk9/4(cfblk11), cfblk10/6(cfblk12)
  cfblk7/1 -> cfblk23/1, cfblk24/1
  cfblk5/1 -> cfblk6/1, cfblk10/5(cfblk11), cfblk26/1
  cfblk11/1(cfblk2) -> cfblk6/2
  cfblk11/2(cfblk13) -> cfblk7/1
  cfblk11/3(cfblk14) -> cfblk4/1
  cfblk9/2(cfblk16) -> cfblk3/1, cfblk20/1
  cfblk8/1(cfblk2) -> cfblk12/1(cfblk1), cfblk10/8(cfblk14)
  cfblk1/1 -> cfblk13/3(cfblk9), cfblk8/4(cfblk8), cfblk12/2(cfblk4)
  cfblk13/1(cfblk2) -> cfblk8/1(cfblk1), cfblk5/1, cfblk11/5(cfblk10)
  cfblk11/4(cfblk15) -> cfblk3/2, cfblk9/7(cfblk14), cfblk27/1
  cfblk12/1(cfblk2) -> cfblk11/2(cfblk7)
  cfblk6/1 -> cfblk10/1(cfblk1), cfblk10/4(cfblk10), cfblk22/1
  cfblk4/1 -> cfblk5/2, cfblk10/3(cfblk9), cfblk9/8(cfblk15), cfblk25/1
  cfblk3/1 -> cfblk2/1, cfblk17/1, cfblk18/1, cfblk19/1
  cfblk12/2(cfblk7) -> cfblk9/1(cfblk1)
  cfblk10/2(cfblk15) -> cfblk9/2(cfblk9)
  cfblk10/3(cfblk16) -> cfblk9/3(cfblk10), cfblk9/5(cfblk12), cfblk9/6(cfblk13), cfblk21/1
  cfblk12/3(cfblk8) -> cfblk11/7(cfblk12), cfblk28/1
  cfblk10/1(cfblk2) -> cfblk15/1
  cfblk15/1 -> cfblk8/2(cfblk6)
  cfblk9/1(cfblk2) -> cfblk16/1
  cfblk16/1 -> cfblk13/2(cfblk8)
  cfblk17/1 -> cfblk10/2(cfblk8)
  cfblk18/1 -> cfblk11/6(cfblk11)
  cfblk19/1 -> cfblk10/7(cfblk13)
  cfblk20/1 -> cfblk13/5(cfblk11)
  cfblk21/1 -> cfblk11/3(cfblk8)
  cfblk22/1 -> cfblk11/4(cfblk9)
  cfblk23/1 -> cfblk13/1(cfblk1)
  cfblk24/1 -> cfblk12/3(cfblk5)
  cfblk25/1 -> cfblk13/4(cfblk10)
  cfblk26/1 -> cfblk8/5(cfblk9)
  cfblk27/1 -> cfblk12/4(cfblk6)
  cfblk28/1 -> cfblk8/3(cfblk7)

== system sampleModel20/cfblk96/cfblk7/cfblk7 ==
  cfblk1 : Inport
  cfblk12 : Inport  Port=2
  cfblk13 : Inport  Port=3
  cfblk14 : Inport  Port=4
  cfblk15 : Inport  Port=5
  cfblk16 : Inport  Port=6
  cfblk10 : Subsystem
  cfblk11 : Subsystem
  cfblk17 : Delay  SampleTime=1
  cfblk18 : Delay  SampleTime=1
  cfblk19 : Delay  SampleTime=1
  cfblk3 : MinMax  Inputs=3
  cfblk4 : Signum
  cfblk5 : Product  Inputs=**
  cfblk6 : Product
  cfblk7 : Product  Inputs=*
  cfblk8 : Sum  Inputs=+
  cfblk9 : simulink/Math Operations/MinMax Running Resettable  Function=min  vinit=0.0
  cfblk2 : Outport
  wires:
  cfblk14/1 -> cfblk11/1(cfblk1)
  cfblk4/1 -> cfblk11/2(cfblk10)
  cfblk15/1 -> cfblk4/1
  cfblk6/1 -> cfblk2/1
  cfblk10/1(cfblk2) -> cfblk8/1
  cfblk3/1 -> cfblk7/1, cfblk10/5(cfblk11)
  cfblk5/1 -> cfblk6/1, cfblk19/1
  cfblk13/1 -> cfblk3/2
  cfblk1/1 -> cfblk9/2
  cfblk7/1 -> cfblk10/1(cfblk1)
  cfblk16/1 -> cfblk5/1
  cfblk10/3(cfblk13) -> cfblk5/2
  cfblk9/1 -> cfblk3/3
  cfblk11/1(cfblk2) -> cfblk6/2
  cfblk12/1 -> cfblk10/2(cfblk8), cfblk10/4(cfblk10)
  cfblk8/1 -> cfblk17/1
  cfblk17/1 -> cfblk9/1
  cfblk10/2(cfblk12) -> cfblk18/1
  cfblk18/1 -> cfblk3/1
  cfblk19/1 -> cfblk10/3(cfblk9)

== system sampleModel20/cfblk96/cfblk7/cfblk8 ==
  cfblk1 : Inport
  cfblk10 : Inport  Port=2
  cfblk11 : Inport  Port=3
  cfblk12 : Inport  Port=4
  cfblk{14..17} (4 alike) : Delay  SampleTime=1
  cfblk3 : simulink/Math Operations/Slider Gain  gain=1  low=0  high=2
  cfblk4 : Polyval  Coefs=[ +2.081618890e-019, -1.441693666e-014, +4.719686976e-010, -8.536869453e-006, +1.621573104e-001, -8.087801117e+001 ]
  cfblk5 : Assignment  DiagnosticForDimensions=Warning  IndexOptions=Index vector (dialog)  Indices=1  OutputSizes=1
  cfblk6 : Sum  Inputs=+-
  cfblk7 : Sum  Inputs=+-
  cfblk8 : Abs
  cfblk9 : Subsystem
  cfblk2 : Outport
  cfblk13 : Outport  Port=2
  wires:
  cfblk9/1(cfblk2) -> cfblk4/1
  cfblk6/1 -> cfblk8/1, cfblk17/1
  cfblk7/1 -> cfblk6/1
  cfblk11/1 -> cfblk6/2, cfblk9/6(cfblk12)
  cfblk10/1 -> cfblk3/1
  cfblk1/1 -> cfblk9/1(cfblk1)
  cfblk9/2(cfblk13) -> cfblk2/1
  cfblk3/1 -> cfblk5/1, cfblk13/1
  cfblk12/1 -> cfblk9/2(cfblk8)
  cfblk4/1 -> cfblk5/2, cfblk15/1
  cfblk9/3(cfblk14) -> cfblk7/2
  cfblk5/1 -> cfblk14/1
  cfblk14/1 -> cfblk9/3(cfblk9)
  cfblk15/1 -> cfblk9/5(cfblk11)
  cfblk8/1 -> cfblk16/1
  cfblk16/1 -> cfblk7/1
  cfblk17/1 -> cfblk9/4(cfblk10)

== system sampleModel20/cfblk97/cfblk3/cfblk10 ==
  cfblk1 : Inport
  cfblk8 : Inport  Port=2
  cfblk9 : Inport  Port=3
  cfblk10 : Inport  Port=4
  cfblk{11..15} (5 alike) : Delay  SampleTime=1
  cfblk3 : Sum  Inputs=+
  cfblk4 : Sin  TimeSource=Use external signal  SampleTime=0
  cfblk5 : MinMax  Inputs=3
  cfblk6 : Subsystem
  cfblk7 : Subsystem
  cfblk2 : Outport
  wires:
  cfblk6/1(cfblk2) -> cfblk3/1
  cfblk9/1 -> cfblk2/1, cfblk6/8(cfblk13)
  cfblk3/1 -> cfblk5/1
  cfblk4/1 -> cfblk11/1, cfblk12/1, cfblk13/1
  cfblk8/1 -> cfblk7/2(cfblk5), cfblk7/5(cfblk8), cfblk6/6(cfblk11), cfblk6/9(cfblk14)
  cfblk10/1 -> cfblk7/3(cfblk6), cfblk6/3(cfblk8)
  cfblk5/1 -> cfblk14/1, cfblk15/1
  cfblk1/1 -> cfblk7/4(cfblk7), cfblk5/2, cfblk6/5(cfblk10)
  cfblk7/1(cfblk2) -> cfblk4/1
  cfblk7/2(cfblk11) -> cfblk6/2(cfblk7), cfblk6/4(cfblk9), cfblk5/3, cfblk6/10(cfblk15), cfblk6/11(cfblk16)
  cfblk11/1 -> cfblk7/1(cfblk1)
  cfblk12/1 -> cfblk7/6(cfblk9)
  cfblk13/1 -> cfblk7/7(cfblk10)
  cfblk14/1 -> cfblk6/1(cfblk1)
  cfblk15/1 -> cfblk6/7(cfblk12)

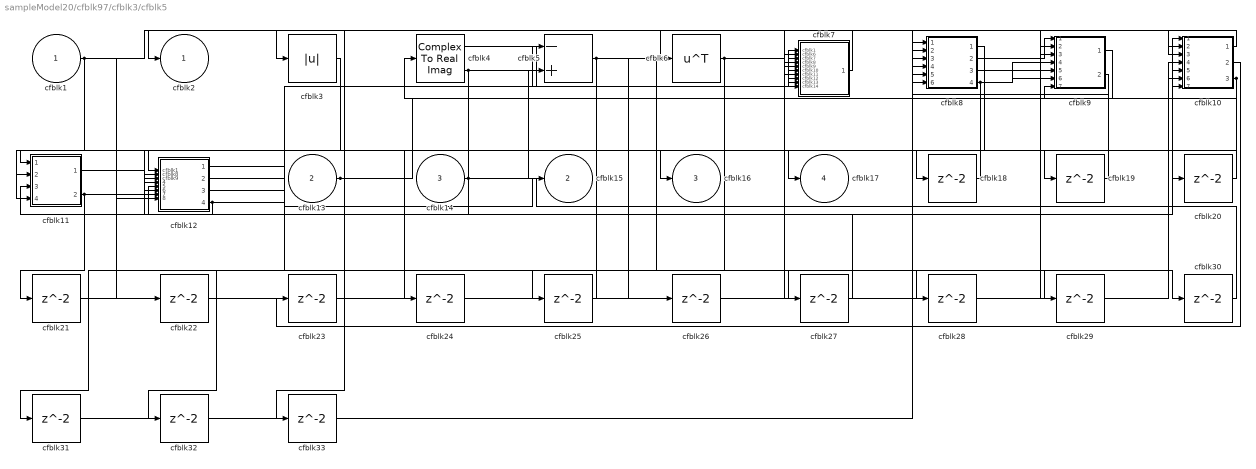
== system sampleModel20/cfblk97/cfblk3/cfblk5 ==
  cfblk1 : Inport
  cfblk13 : Inport  Port=2
  cfblk14 : Inport  Port=3
  cfblk10 : Subsystem
  cfblk11 : Subsystem
  cfblk12 : Subsystem
  cfblk{18..33} (16 alike) : Delay  SampleTime=1
  cfblk3 : Abs
  cfblk4 : ComplexToRealImag
  cfblk5 : Sum  Inputs=-+
  cfblk6 : Math  Operator=transpose  SaturateOnIntegerOverflow=on
  cfblk7 : Subsystem
  cfblk8 : Subsystem
  cfblk9 : Subsystem
  cfblk2 : Outport
  cfblk15 : Outport  Port=2
  cfblk16 : Outport  Port=3
  cfblk17 : Outport  Port=4
  wires:
  cfblk3/1 -> cfblk11/1(cfblk1)
  cfblk13/1 -> cfblk2/1, cfblk10/5(cfblk11)
  cfblk10/1(cfblk2) -> cfblk3/1
  cfblk9/1(cfblk2) -> cfblk4/1
  cfblk4/1 -> cfblk7/1(cfblk1)
  cfblk9/2(cfblk14) -> cfblk12/1(cfblk1)
  cfblk6/1 -> cfblk16/1, cfblk10/3(cfblk9), cfblk10/7(cfblk13), cfblk18/1, cfblk31/1, cfblk32/1
  cfblk7/1(cfblk2) -> cfblk6/1
  cfblk11/2(cfblk9) -> cfblk20/1, cfblk21/1, cfblk22/1
  cfblk8/1(cfblk2) -> cfblk17/1
  cfblk14/1 -> cfblk10/1(cfblk1), cfblk12/3(cfblk9), cfblk12/5(cfblk11), cfblk7/6(cfblk10), cfblk9/7(cfblk13), cfblk7/9(cfblk13)
  cfblk4/2 -> cfblk7/3(cfblk7), cfblk7/8(cfblk12), cfblk33/1
  cfblk10/3(cfblk15) -> cfblk12/4(cfblk10), cfblk24/1
  cfblk12/1(cfblk2) -> cfblk5/1
  cfblk8/2(cfblk13) -> cfblk9/1(cfblk1)
  cfblk1/1 -> cfblk8/3(cfblk9), cfblk12/8(cfblk14), cfblk11/4(cfblk8), cfblk9/5(cfblk11)
  cfblk8/3(cfblk14) -> cfblk10/2(cfblk8)
  cfblk5/1 -> cfblk25/1, cfblk26/1, cfblk27/1
  cfblk8/4(cfblk15) -> cfblk11/2(cfblk6), cfblk12/7(cfblk13), cfblk9/4(cfblk10), cfblk9/6(cfblk12)
  cfblk12/2(cfblk15) -> cfblk15/1
  cfblk12/3(cfblk16) -> cfblk5/2
  cfblk12/4(cfblk17) -> cfblk11/3(cfblk7), cfblk28/1, cfblk29/1, cfblk30/1
  cfblk18/1 -> cfblk7/5(cfblk9)
  cfblk11/1(cfblk2) -> cfblk19/1
  cfblk19/1 -> cfblk8/1(cfblk1)
  cfblk20/1 -> cfblk7/2(cfblk6)
  cfblk21/1 -> cfblk9/3(cfblk9)
  cfblk22/1 -> cfblk7/10(cfblk14)
  cfblk10/2(cfblk14) -> cfblk23/1
  cfblk23/1 -> cfblk7/4(cfblk8)
  cfblk24/1 -> cfblk8/2(cfblk8)
  cfblk25/1 -> cfblk12/2(cfblk8)
  cfblk26/1 -> cfblk10/4(cfblk10)
  cfblk27/1 -> cfblk12/6(cfblk12)
  cfblk28/1 -> cfblk9/2(cfblk8)
  cfblk29/1 -> cfblk10/6(cfblk12)
  cfblk30/1 -> cfblk7/7(cfblk11)
  cfblk31/1 -> cfblk8/5(cfblk11)
  cfblk32/1 -> cfblk8/6(cfblk12)
  cfblk33/1 -> cfblk8/4(cfblk10)

== system sampleModel20/cfblk97/cfblk3/cfblk6 ==
  cfblk1 : Inport
  cfblk13 : Inport  Port=2
  cfblk10 : Subsystem
  cfblk11 : Subsystem
  cfblk12 : Subsystem
  cfblk{15..20} (6 alike) : Delay  SampleTime=1
  cfblk3 : simulink/Math Operations/Slider Gain  gain=1  low=0  high=2
  cfblk4 : Product  Inputs=**
  cfblk5 : Rounding
  cfblk6 : Trigonometry
  cfblk7 : MinMax
  cfblk8 : Subsystem
  cfblk9 : Subsystem
  cfblk2 : Outport
  cfblk14 : Outport  Port=2
  wires:
  cfblk1/1 -> cfblk5/1, cfblk10/4(cfblk6)
  cfblk5/1 -> cfblk6/1, cfblk3/1
  cfblk12/1(cfblk2) -> cfblk10/6(cfblk8), cfblk15/1
  cfblk13/1 -> cfblk4/1, cfblk10/1(cfblk1), cfblk10/3(cfblk5)
  cfblk4/1 -> cfblk9/1(cfblk1), cfblk20/1
  cfblk11/1(cfblk2) -> cfblk8/1(cfblk1)
  cfblk11/2(cfblk12) -> cfblk4/2
  cfblk9/1(cfblk2) -> cfblk2/1
  cfblk3/1 -> cfblk8/2(cfblk5), cfblk12/2(cfblk6)
  cfblk10/1(cfblk2) -> cfblk16/1, cfblk17/1, cfblk18/1
  cfblk7/1 -> cfblk9/2(cfblk10), cfblk10/2(cfblk4), cfblk8/3(cfblk6), cfblk10/5(cfblk7)
  cfblk9/2(cfblk13) -> cfblk12/1(cfblk1)
  cfblk11/3(cfblk13) -> cfblk7/1, cfblk12/4(cfblk8), cfblk10/7(cfblk9)
  cfblk9/3(cfblk14) -> cfblk14/1, cfblk12/3(cfblk7), cfblk19/1
  cfblk8/1(cfblk2) -> cfblk9/3(cfblk11)
  cfblk6/1 -> cfblk11/3(cfblk9), cfblk12/5(cfblk9)
  cfblk15/1 -> cfblk11/1(cfblk1)
  cfblk16/1 -> cfblk11/2(cfblk8)
  cfblk17/1 -> cfblk9/4(cfblk12)
  cfblk18/1 -> cfblk8/4(cfblk7)
  cfblk19/1 -> cfblk11/4(cfblk10)
  cfblk20/1 -> cfblk11/5(cfblk11)

== system sampleModel20/cfblk97/cfblk3/cfblk7 ==
  cfblk1 : Inport
  cfblk7 : Inport  Port=2
  cfblk{9..13} (5 alike) : Delay  SampleTime=1
  cfblk3 : Assignment  DiagnosticForDimensions=Warning  IndexOptions=Index vector (dialog)  Indices=1  OutputSizes=1
  cfblk4 : Sin  TimeSource=Use external signal  SampleTime=0
  cfblk5 : Subsystem
  cfblk6 : Subsystem
  cfblk2 : Outport
  cfblk8 : Outport  Port=2
  wires:
  cfblk3/1 -> cfblk8/1, cfblk9/1, cfblk10/1
  cfblk1/1 -> cfblk6/1(cfblk1), cfblk5/3(cfblk9)
  cfblk7/1 -> cfblk5/1(cfblk1), cfblk6/2(cfblk7), cfblk6/7(cfblk12)
  cfblk6/1(cfblk2) -> cfblk4/1
  cfblk4/1 -> cfblk2/1, cfblk5/2(cfblk8), cfblk5/4(cfblk10)
  cfblk5/1(cfblk2) -> cfblk3/1
  cfblk5/2(cfblk12) -> cfblk3/2, cfblk11/1, cfblk12/1, cfblk13/1
  cfblk9/1 -> cfblk6/6(cfblk11)
  cfblk10/1 -> cfblk5/5(cfblk11)
  cfblk11/1 -> cfblk6/3(cfblk8)
  cfblk12/1 -> cfblk6/4(cfblk9)
  cfblk13/1 -> cfblk6/5(cfblk10)

== system sampleModel20/cfblk97/cfblk3/cfblk8 ==
  cfblk1 : Inport
  cfblk7 : Inport  Port=2
  cfblk{9..13} (5 alike) : Delay  SampleTime=1
  cfblk3 : Product
  cfblk4 : Sqrt  Operator=rSqrt  AlgorithmType=Newton-Raphson  SaturateOnIntegerOverflow=on
  cfblk5 : Subsystem
  cfblk6 : Subsystem
  cfblk2 : Outport
  cfblk8 : Outport  Port=2
  wires:
  cfblk1/1 -> cfblk2/1, cfblk3/2, cfblk6/4(cfblk11), cfblk5/6(cfblk13), cfblk5/7(cfblk14), cfblk6/7(cfblk14)
  cfblk5/1(cfblk2) -> cfblk8/1
  cfblk6/1(cfblk2) -> cfblk5/1(cfblk1), cfblk5/4(cfblk11), cfblk5/5(cfblk12)
  cfblk5/2(cfblk16) -> cfblk4/1, cfblk13/1
  cfblk3/1 -> cfblk6/1(cfblk1), cfblk6/5(cfblk12)
  cfblk4/1 -> cfblk9/1, cfblk10/1, cfblk11/1, cfblk12/1
  cfblk7/1 -> cfblk5/3(cfblk10), cfblk6/6(cfblk13)
  cfblk9/1 -> cfblk5/2(cfblk9)
  cfblk10/1 -> cfblk6/2(cfblk9)
  cfblk11/1 -> cfblk6/3(cfblk10)
  cfblk12/1 -> cfblk5/8(cfblk15)
  cfblk13/1 -> cfblk3/1

== system sampleModel20/cfblk97/cfblk3/cfblk9 ==
  cfblk1 : Inport
  cfblk14 : Inport  Port=2
  cfblk15 : Inport  Port=3
  cfblk10 : Subsystem
  cfblk11 : Subsystem
  cfblk12 : Subsystem
  cfblk13 : Subsystem
  cfblk{18..21} (4 alike) : Delay  SampleTime=1
  cfblk3 : Math  Operator=magnitude^2  SaturateOnIntegerOverflow=on
  cfblk4 : Squeeze
  cfblk5 : Reshape
  cfblk6 : simulink/Math Operations/Slider Gain  gain=1  low=0  high=2
  cfblk7 : Sin  TimeSource=Use external signal  SampleTime=0
  cfblk8 : Squeeze
  cfblk9 : Assignment  DiagnosticForDimensions=Warning  IndexOptions=Index vector (dialog)  Indices=1  OutputSizes=1
  cfblk2 : Outport
  cfblk16 : Outport  Port=2
  cfblk17 : Outport  Port=3
  wires:
  cfblk12/1(cfblk2) -> cfblk4/1
  cfblk9/1 -> cfblk3/1
  cfblk11/1(cfblk2) -> cfblk9/1, cfblk10/3(cfblk11), cfblk20/1
  cfblk14/1 -> cfblk12/1(cfblk1)
  cfblk6/1 -> cfblk10/1(cfblk1)
  cfblk13/1(cfblk2) -> cfblk7/1
  cfblk3/1 -> cfblk2/1, cfblk17/1
  cfblk7/1 -> cfblk18/1, cfblk19/1
  cfblk10/1(cfblk2) -> cfblk8/1
  cfblk15/1 -> cfblk5/1, cfblk13/1(cfblk1)
  cfblk12/2(cfblk13) -> cfblk11/1(cfblk1)
  cfblk4/1 -> cfblk9/2, cfblk13/2(cfblk8)
  cfblk8/1 -> cfblk16/1, cfblk21/1
  cfblk1/1 -> cfblk12/3(cfblk8), cfblk12/4(cfblk9)
  cfblk13/2(cfblk9) -> cfblk11/2(cfblk8)
  cfblk5/1 -> cfblk6/1, cfblk10/4(cfblk12)
  cfblk13/3(cfblk10) -> cfblk10/2(cfblk10)
  cfblk18/1 -> cfblk12/2(cfblk7)
  cfblk19/1 -> cfblk12/6(cfblk11)
  cfblk20/1 -> cfblk12/5(cfblk10)
  cfblk21/1 -> cfblk12/7(cfblk12)
